simulink model "timeSharedStat"  (R2025a)
settings: Solver=VariableStepAuto  StartTime=0.0  StopTime=10.0  RelTol=1e-3
libraries: StdLib x15, TimeSharedLib x2
settings Model: Creator=peter  LastModifiedBy=peter
settings RTWCC: GPUComputeCapability=3.5

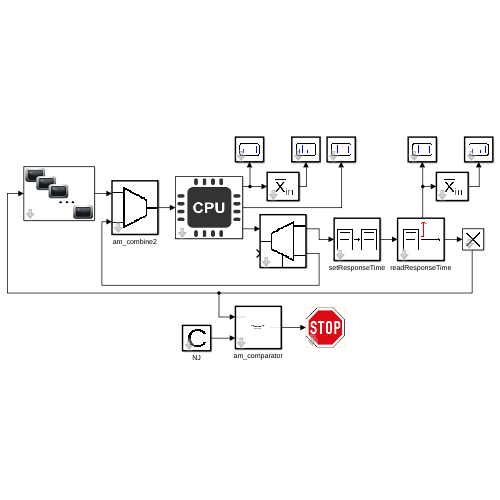
[thumbnail: Simulink's stored preview of the top-level diagram]
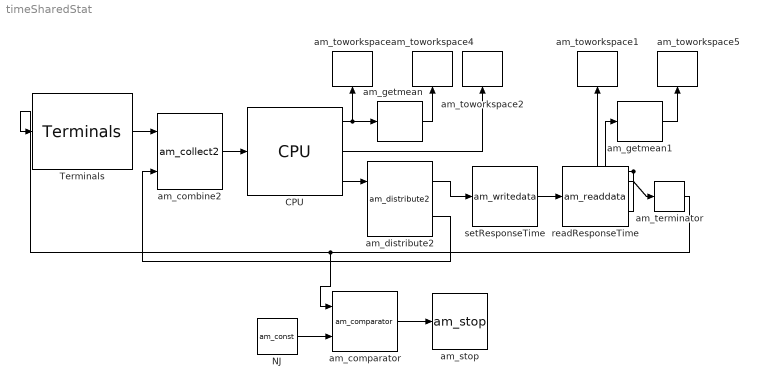
== system timeSharedStat ==
  CPU : TimeSharedLib/CPU  q=0.1  tSwap=0.015
  NJ : StdLib/am_const  value=1000  sendTime=[0,1]  debug=0
  Terminals : TimeSharedLib/Terminals  N=80  tW=25  tS=0.8
  am_combine2 : StdLib/am_collect2  tD=[0,2]  tau=[0,1]  debug=0
  am_comparator : StdLib/am_comparator  compop="\"==\""  tau=[0,1]  debug=0
  am_distribute2 : StdLib/am_distribute2  port0=1  field="\"outPort\""  tau=[0,1]  debug=0
  am_getmean : StdLib/am_getmean  tau=[0,1]  debug=0
  am_getmean1 : StdLib/am_getmean  tau=[0,1]  debug=0
  am_stop : StdLib/am_stop  tau=[0,1]  debug=0
  am_terminator : StdLib/am_terminator  tau=[0,1]  debug=0
  am_toworkspace : StdLib/am_toworkspace  varname="\"nQ\""  t0=0  format="\"vector\""  tau=[0,5]  debug=0
  am_toworkspace1 : StdLib/am_toworkspace  varname="\"tR\""  t0=0  format="\"vector\""  tau=[0,1]  debug=0
  am_toworkspace2 : StdLib/am_toworkspace  varname="\"util\""  t0=0  format="\"vector\""  tau=[0,5]  debug=0
  am_toworkspace4 : StdLib/am_toworkspace  varname="\"nQMean\""  t0=0  format="\"vector\""  tau=[0,5]  debug=0
  am_toworkspace5 : StdLib/am_toworkspace  varname="\"tRMean\""  t0=0  format="\"vector\""  tau=[0,1]  debug=0
  readResponseTime : StdLib/am_readdata  field="\"startTime\""  tau=[0,1]  debug=0
  setResponseTime : StdLib/am_writedata  inFields="\"startTime\""  outField="\"startTime\""  changeFunc="\"out = get_time() - in(1);\""  tau=[0,1]  debug=0
  wires:
  Terminals/1 -> am_combine2/1
  am_combine2/1 -> CPU/1
  CPU/3 -> am_distribute2/1
  am_distribute2/1 -> setResponseTime/1
  am_distribute2/2 -> am_combine2/2
  am_terminator/1 -> am_comparator/1, Terminals/1
  CPU/1 -> am_toworkspace/1, am_getmean/1
  am_comparator/1 -> am_stop/1
  NJ/1 -> am_comparator/2
  readResponseTime/1 -> am_terminator/1
  readResponseTime/2 -> am_toworkspace1/1, am_getmean1/1
  setResponseTime/1 -> readResponseTime/1
  CPU/2 -> am_toworkspace2/1
  am_getmean/1 -> am_toworkspace4/1
  am_getmean1/1 -> am_toworkspace5/1
